simulink model "SolarTrackerSimulationModel"  (R2020a)
settings: Solver=FixedStepAuto  StartTime=0.0  StopTime=inf  RelTol=1e-3
libraries: sldrtlib x9, simulink x2
settings Model: SILPILModeSetting=veronly  EnablePacing=on  ExtModeTrigDuration=2  Creator=cstap  LastModifiedBy=dbhatia
settings OptimizationCC: EnhancedBackFolding=on  PassReuseOutputArgsAs=Individual arguments  ZeroExternalMemoryAtStartup=off  ZeroInternalMemoryAtStartup=off  MaxStackSize=64  OptimizeBlockOrder=speed  DifferentSizesBufferReuse=on  OptimizationCustomize=off  EfficientTunableParamExpr=on
settings DebuggingCC: ParameterTunabilityLossMsg=error
settings HardwareCC: ProdBitPerPointer=32  ProdBitPerSizeT=32  ProdBitPerPtrDiffT=32  ProdLargestAtomicInteger=Long  ProdLargestAtomicFloat=Double  ProdWordSize=32  ProdHWDeviceType=ARM Compatible->ARM Cortex
settings SFSimCC: MATLABDynamicMemAlloc=off
settings RTWCC: SystemTargetFile=ert.tlc  HardwareBoard=Arduino MKR1000  TLCOptions=-aInlineSetEventsForThisBaseRateFcn=TLC_FALSE -aSuppressMultiTaskScheduler=TLC_FALSE -aRateBasedStepFcn=1  TemplateMakefile=ert_default_tmf  Toolchain=Arduino ARM  BuildConfiguration=Faster Runs
settings CodeAppCC: ForceParamTrailComments=on  IgnoreCustomStorageClasses=off  OperatorAnnotations=on  SimulinkDataObjDesc=on  SFDataObjDesc=on  InsertBlockDesc=on
settings ERTTargetCC: SupportContinuousTime=on  SupportVariableSizeSignals=on  ExtModeStaticAllocSize=8192

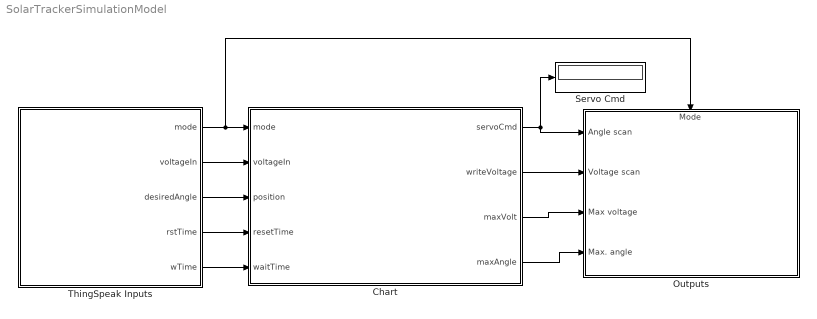
== system SolarTrackerSimulationModel ==
  Chart : Stateflow chart  TreatAsAtomicUnit=on
      settings: PortSchema="{\"entries\":[{\"content\":{\"sides\":[{\"content\":{\"connectorIds\":[\"In5\",\"In1\",\"In2\",\"In3\",\"In4\"]},\"type\":\"ConnectorPlacement.EquallySpacedRectSide\",\"uuid\":\"7460febf-f6e8-4dab-9ef6-8acf957c7b17\"},{\"content\":{\"connectorIds\":[\"Out1\",\"Out2\",\"Out3\",\"Out4\"],\"side\":\"RIGHT\"},\"type\":\"ConnectorPlacement.EquallySpacedRectSide\",\"uuid\":\"34f4fde0-3abd-4f83-b5ac-d115b7860e10\"},{\"content\":{\"connectorIds\":[],\"side\":\"TOP\"},\"type\":\"ConnectorPlacement.EquallySpacedRectSide\",\"uuid\":\"03c52414-b361-422d-a974-9760757eaedc\"}]},\"type\":\"ConnectorPlacement.EquallySpacedConnector\",\"uuid\":\"cf5b2fd0-3883-4494-a5b1-8c312db57bd7\"}],\"packageUris\":[\"http://schema.mathworks.com/mf0/Connector/19700101\"],\"version\":\"1.0\"}"
  Outputs : Subsystem
      settings: PortSchema="{\"entries\":[{\"content\":{\"sides\":[{\"content\":{\"connectorIds\":[\"In1\",\"In2\",\"In3\",\"In4\"]},\"type\":\"ConnectorPlacement.EquallySpacedRectSide\",\"uuid\":\"80b3db40-b16c-4fd7-bc95-d011d1dc8e0f\"},{\"content\":{\"connectorIds\":[],\"side\":\"RIGHT\"},\"type\":\"ConnectorPlacement.EquallySpacedRectSide\",\"uuid\":\"c08e910d-1728-45ea-85cd-9044765ba3b0\"},{\"content\":{\"connectorIds\":[\"In5\"],\"side\":\"TOP\"},\"type\":\"ConnectorPlacement.EquallySpacedRectSide\",\"uuid\":\"a6fb2687-566e-4921-9db4-7b726284379e\"}]},\"type\":\"ConnectorPlacement.EquallySpacedConnector\",\"uuid\":\"da0eea2f-bb34-402a-a1e4-ed3247ba3f26\"}],\"packageUris\":[\"http://schema.mathworks.com/mf0/Connector/19700101\"],\"version\":\"1.0\"}"
  Servo Cmd : Display
  ThingSpeak Inputs : Subsystem
  wires:
  ThingSpeak Inputs/1(mode) -> Outputs/5(Mode), Chart/5(mode)
  ThingSpeak Inputs/2(voltageIn) -> Chart/1(voltageIn)
  ThingSpeak Inputs/3(desiredAngle) -> Chart/2(position)
  ThingSpeak Inputs/4(rstTime) -> Chart/3(resetTime)
  ThingSpeak Inputs/5(wTime) -> Chart/4(waitTime)
  Chart/2(writeVoltage) -> Outputs/2(Voltage scan)
  Chart/3(maxVolt) -> Outputs/3(Max voltage)
  Chart/4(maxAngle) -> Outputs/4(Max. angle)
  Chart/1(servoCmd) -> Outputs/1(Angle scan), Servo Cmd/1

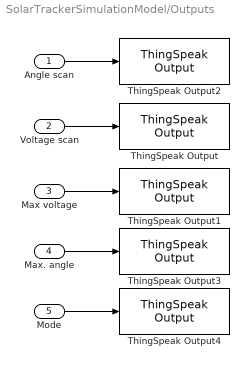
== system SolarTrackerSimulationModel/Outputs ==
  Angle scan : Inport
  Voltage scan : Inport  Port=2
  Max voltage : Inport  Port=3
  Max. angle : Inport  Port=4
  Mode : Inport  Port=5
  ThingSpeak Output : sldrtlib/Internet of Things/ThingSpeak Output  DrvAddress=1049171  DrvOptions=[1 10 77 88 84 86 78 50 89 78 70 66 88 88 75 72 71 55 97 112 105 46 116 104 105 110 103 115 112 101 97 107 46 99 111 109 0 0 0 0 0 0 0 0 0 0 0 0 0 0 0 0 0 0 0 0 0 0 0 0 0 0 0 0 0 0 0 0 0 0 0 0 0 0 0 0 0 0 0 0 0 0 0 0 0 0 0 0 0 0 0 0 0 0 0 0 0 0 0 0 0 0 0 0 0 0 0 0 0 0 0 0 0 0 0 0 0 0 0 0 0 0 0 0 0 0 0 0 0 0 0 0 0 0 0 0 0 0 0 0 0 0 0 0 0 0 0 0 0 0 0 0 0 0 0 0 0 0 0 0 0 0 0 0 0 0 0 0 0 0 0 0 0 0 0 0 0 0 0 0 0 0 0 0 0 0 0 0 0 0 0 0 0 0 0 0 0 0 0 0 0 0 0 0 0 0 0 0 0 0 0 0 0 0 0 0 0 0 0 0 0 0 0 0 0 0 0 0 0 0 0 0 0 0 0 0 0 0 0 0 0 0 0 0 0 0 0 0 0 0 0 0 0 0 0 0]  SampleTime=15  MaxMissedTicks=10  ShowMissedTicks=off  YieldWhenWaiting=off  ChannelFields=1  OptParam=0  InitialValue=[]  FinalValue=[]
      settings: SourceProductBaseCode=WT
  ThingSpeak Output1 : sldrtlib/Internet of Things/ThingSpeak Output  DrvAddress=1049171  DrvOptions=[1 10 77 88 84 86 78 50 89 78 70 66 88 88 75 72 71 55 97 112 105 46 116 104 105 110 103 115 112 101 97 107 46 99 111 109 0 0 0 0 0 0 0 0 0 0 0 0 0 0 0 0 0 0 0 0 0 0 0 0 0 0 0 0 0 0 0 0 0 0 0 0 0 0 0 0 0 0 0 0 0 0 0 0 0 0 0 0 0 0 0 0 0 0 0 0 0 0 0 0 0 0 0 0 0 0 0 0 0 0 0 0 0 0 0 0 0 0 0 0 0 0 0 0 0 0 0 0 0 0 0 0 0 0 0 0 0 0 0 0 0 0 0 0 0 0 0 0 0 0 0 0 0 0 0 0 0 0 0 0 0 0 0 0 0 0 0 0 0 0 0 0 0 0 0 0 0 0 0 0 0 0 0 0 0 0 0 0 0 0 0 0 0 0 0 0 0 0 0 0 0 0 0 0 0 0 0 0 0 0 0 0 0 0 0 0 0 0 0 0 0 0 0 0 0 0 0 0 0 0 0 0 0 0 0 0 0 0 0 0 0 0 0 0 0 0 0 0 0 0 0 0 0 0 0 0]  SampleTime=15  MaxMissedTicks=10  ShowMissedTicks=off  YieldWhenWaiting=off  ChannelFields=3  OptParam=0  InitialValue=[]  FinalValue=[]
      settings: SourceProductBaseCode=WT
  ThingSpeak Output2 : sldrtlib/Internet of Things/ThingSpeak Output  DrvAddress=1049171  DrvOptions=[1 10 77 88 84 86 78 50 89 78 70 66 88 88 75 72 71 55 97 112 105 46 116 104 105 110 103 115 112 101 97 107 46 99 111 109 0 0 0 0 0 0 0 0 0 0 0 0 0 0 0 0 0 0 0 0 0 0 0 0 0 0 0 0 0 0 0 0 0 0 0 0 0 0 0 0 0 0 0 0 0 0 0 0 0 0 0 0 0 0 0 0 0 0 0 0 0 0 0 0 0 0 0 0 0 0 0 0 0 0 0 0 0 0 0 0 0 0 0 0 0 0 0 0 0 0 0 0 0 0 0 0 0 0 0 0 0 0 0 0 0 0 0 0 0 0 0 0 0 0 0 0 0 0 0 0 0 0 0 0 0 0 0 0 0 0 0 0 0 0 0 0 0 0 0 0 0 0 0 0 0 0 0 0 0 0 0 0 0 0 0 0 0 0 0 0 0 0 0 0 0 0 0 0 0 0 0 0 0 0 0 0 0 0 0 0 0 0 0 0 0 0 0 0 0 0 0 0 0 0 0 0 0 0 0 0 0 0 0 0 0 0 0 0 0 0 0 0 0 0 0 0 0 0 0 0]  SampleTime=15  MaxMissedTicks=10  ShowMissedTicks=off  YieldWhenWaiting=off  ChannelFields=2  OptParam=0  InitialValue=[]  FinalValue=[]
      settings: SourceProductBaseCode=WT
  ThingSpeak Output3 : sldrtlib/Internet of Things/ThingSpeak Output  DrvAddress=1049171  DrvOptions=[1 10 77 88 84 86 78 50 89 78 70 66 88 88 75 72 71 55 97 112 105 46 116 104 105 110 103 115 112 101 97 107 46 99 111 109 0 0 0 0 0 0 0 0 0 0 0 0 0 0 0 0 0 0 0 0 0 0 0 0 0 0 0 0 0 0 0 0 0 0 0 0 0 0 0 0 0 0 0 0 0 0 0 0 0 0 0 0 0 0 0 0 0 0 0 0 0 0 0 0 0 0 0 0 0 0 0 0 0 0 0 0 0 0 0 0 0 0 0 0 0 0 0 0 0 0 0 0 0 0 0 0 0 0 0 0 0 0 0 0 0 0 0 0 0 0 0 0 0 0 0 0 0 0 0 0 0 0 0 0 0 0 0 0 0 0 0 0 0 0 0 0 0 0 0 0 0 0 0 0 0 0 0 0 0 0 0 0 0 0 0 0 0 0 0 0 0 0 0 0 0 0 0 0 0 0 0 0 0 0 0 0 0 0 0 0 0 0 0 0 0 0 0 0 0 0 0 0 0 0 0 0 0 0 0 0 0 0 0 0 0 0 0 0 0 0 0 0 0 0 0 0 0 0 0 0]  SampleTime=15  MaxMissedTicks=10  ShowMissedTicks=off  YieldWhenWaiting=off  ChannelFields=4  OptParam=0  InitialValue=[]  FinalValue=[]
      settings: SourceProductBaseCode=WT
  ThingSpeak Output4 : sldrtlib/Internet of Things/ThingSpeak Output  DrvAddress=1049171  DrvOptions=[1 10 77 88 84 86 78 50 89 78 70 66 88 88 75 72 71 55 97 112 105 46 116 104 105 110 103 115 112 101 97 107 46 99 111 109 0 0 0 0 0 0 0 0 0 0 0 0 0 0 0 0 0 0 0 0 0 0 0 0 0 0 0 0 0 0 0 0 0 0 0 0 0 0 0 0 0 0 0 0 0 0 0 0 0 0 0 0 0 0 0 0 0 0 0 0 0 0 0 0 0 0 0 0 0 0 0 0 0 0 0 0 0 0 0 0 0 0 0 0 0 0 0 0 0 0 0 0 0 0 0 0 0 0 0 0 0 0 0 0 0 0 0 0 0 0 0 0 0 0 0 0 0 0 0 0 0 0 0 0 0 0 0 0 0 0 0 0 0 0 0 0 0 0 0 0 0 0 0 0 0 0 0 0 0 0 0 0 0 0 0 0 0 0 0 0 0 0 0 0 0 0 0 0 0 0 0 0 0 0 0 0 0 0 0 0 0 0 0 0 0 0 0 0 0 0 0 0 0 0 0 0 0 0 0 0 0 0 0 0 0 0 0 0 0 0 0 0 0 0 0 0 0 0 0 0]  SampleTime=15  MaxMissedTicks=10  ShowMissedTicks=off  YieldWhenWaiting=off  ChannelFields=5  OptParam=0  InitialValue=[]  FinalValue=[]
      settings: SourceProductBaseCode=WT
  wires:
  Voltage scan/1 -> ThingSpeak Output/1
  Angle scan/1 -> ThingSpeak Output2/1
  Max voltage/1 -> ThingSpeak Output1/1
  Max. angle/1 -> ThingSpeak Output3/1
  Mode/1 -> ThingSpeak Output4/1

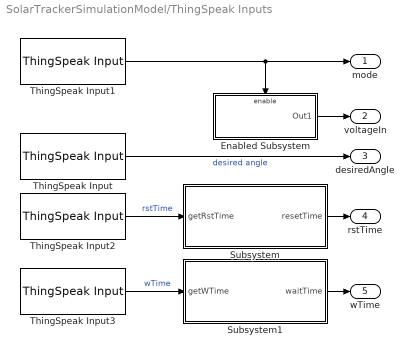
== system SolarTrackerSimulationModel/ThingSpeak Inputs ==
  Enabled Subsystem : Subsystem  TreatAsAtomicUnit=on
  Subsystem : Subsystem
  Subsystem1 : Subsystem
  ThingSpeak Input : sldrtlib/Internet of Things/ThingSpeak Input  DrvAddress=1049139  DrvOptions=[0 1 84 52 67 75 85 73 73 71 66 66 69 84 80 70 66 68 97 112 105 46 116 104 105 110 103 115 112 101 97 107 46 99 111 109 0 0 0 0 0 0 0 0 0 0 0 0 0 0 0 0 0 0 0 0 0 0 0 0 0 0 0 0 0 0 0 0 0 0 0 0 0 0 0 0 0 0 0 0 0 0 0 0 0 0 0 0 0 0 0 0 0 0 0 0 0 0 0 0 0 0 0 0 0 0 0 0 0 0 0 0 0 0 0 0 0 0 0 0 0 0 0 0 0 0 0 0 0 0 0 0 0 0 0 0 0 0 0 0 0 0 0 0 0 0 0 0 0 0 0 0 0 0 0 0 0 0 0 0 0 0 0 0 0 0 0 0 0 0 0 0 0 0 0 0 0 0 0 0 0 0 0 0 0 0 0 0 0 0 0 0 0 0 0 0 0 0 0 0 0 0 0 0 0 0 0 0 0 0 0 0 0 0 0 0 0 0 0 0 0 0 0 0 0 0 0 0 0 0 0 0 0 0 0 0 0 0 0 0 0 0 0 0 0 0 0 0 0 0 0 0 0 0 0 0]  SampleTime=0  MaxMissedTicks=10  ShowMissedTicks=off  YieldWhenWaiting=off  ChannelFields=2  OptParam=0  DataTypeStr=double
      settings: SourceProductBaseCode=WT
  ThingSpeak Input1 : sldrtlib/Internet of Things/ThingSpeak Input  DrvAddress=1049139  DrvOptions=[0 1 84 52 67 75 85 73 73 71 66 66 69 84 80 70 66 68 97 112 105 46 116 104 105 110 103 115 112 101 97 107 46 99 111 109 0 0 0 0 0 0 0 0 0 0 0 0 0 0 0 0 0 0 0 0 0 0 0 0 0 0 0 0 0 0 0 0 0 0 0 0 0 0 0 0 0 0 0 0 0 0 0 0 0 0 0 0 0 0 0 0 0 0 0 0 0 0 0 0 0 0 0 0 0 0 0 0 0 0 0 0 0 0 0 0 0 0 0 0 0 0 0 0 0 0 0 0 0 0 0 0 0 0 0 0 0 0 0 0 0 0 0 0 0 0 0 0 0 0 0 0 0 0 0 0 0 0 0 0 0 0 0 0 0 0 0 0 0 0 0 0 0 0 0 0 0 0 0 0 0 0 0 0 0 0 0 0 0 0 0 0 0 0 0 0 0 0 0 0 0 0 0 0 0 0 0 0 0 0 0 0 0 0 0 0 0 0 0 0 0 0 0 0 0 0 0 0 0 0 0 0 0 0 0 0 0 0 0 0 0 0 0 0 0 0 0 0 0 0 0 0 0 0 0 0]  SampleTime=0  MaxMissedTicks=10  ShowMissedTicks=off  YieldWhenWaiting=off  ChannelFields=1  OptParam=0  DataTypeStr=double
      settings: SourceProductBaseCode=WT
  ThingSpeak Input2 : sldrtlib/Internet of Things/ThingSpeak Input  DrvAddress=1049139  DrvOptions=[0 1 84 52 67 75 85 73 73 71 66 66 69 84 80 70 66 68 97 112 105 46 116 104 105 110 103 115 112 101 97 107 46 99 111 109 0 0 0 0 0 0 0 0 0 0 0 0 0 0 0 0 0 0 0 0 0 0 0 0 0 0 0 0 0 0 0 0 0 0 0 0 0 0 0 0 0 0 0 0 0 0 0 0 0 0 0 0 0 0 0 0 0 0 0 0 0 0 0 0 0 0 0 0 0 0 0 0 0 0 0 0 0 0 0 0 0 0 0 0 0 0 0 0 0 0 0 0 0 0 0 0 0 0 0 0 0 0 0 0 0 0 0 0 0 0 0 0 0 0 0 0 0 0 0 0 0 0 0 0 0 0 0 0 0 0 0 0 0 0 0 0 0 0 0 0 0 0 0 0 0 0 0 0 0 0 0 0 0 0 0 0 0 0 0 0 0 0 0 0 0 0 0 0 0 0 0 0 0 0 0 0 0 0 0 0 0 0 0 0 0 0 0 0 0 0 0 0 0 0 0 0 0 0 0 0 0 0 0 0 0 0 0 0 0 0 0 0 0 0 0 0 0 0 0 0]  SampleTime=0  MaxMissedTicks=10  ShowMissedTicks=off  YieldWhenWaiting=off  ChannelFields=3  OptParam=0  DataTypeStr=double
      settings: SourceProductBaseCode=WT
  ThingSpeak Input3 : sldrtlib/Internet of Things/ThingSpeak Input  DrvAddress=1049139  DrvOptions=[0 1 84 52 67 75 85 73 73 71 66 66 69 84 80 70 66 68 97 112 105 46 116 104 105 110 103 115 112 101 97 107 46 99 111 109 0 0 0 0 0 0 0 0 0 0 0 0 0 0 0 0 0 0 0 0 0 0 0 0 0 0 0 0 0 0 0 0 0 0 0 0 0 0 0 0 0 0 0 0 0 0 0 0 0 0 0 0 0 0 0 0 0 0 0 0 0 0 0 0 0 0 0 0 0 0 0 0 0 0 0 0 0 0 0 0 0 0 0 0 0 0 0 0 0 0 0 0 0 0 0 0 0 0 0 0 0 0 0 0 0 0 0 0 0 0 0 0 0 0 0 0 0 0 0 0 0 0 0 0 0 0 0 0 0 0 0 0 0 0 0 0 0 0 0 0 0 0 0 0 0 0 0 0 0 0 0 0 0 0 0 0 0 0 0 0 0 0 0 0 0 0 0 0 0 0 0 0 0 0 0 0 0 0 0 0 0 0 0 0 0 0 0 0 0 0 0 0 0 0 0 0 0 0 0 0 0 0 0 0 0 0 0 0 0 0 0 0 0 0 0 0 0 0 0 0]  SampleTime=0  MaxMissedTicks=10  ShowMissedTicks=off  YieldWhenWaiting=off  ChannelFields=4  OptParam=0  DataTypeStr=double
      settings: SourceProductBaseCode=WT
  mode : Outport
  voltageIn : Outport  Port=2
  desiredAngle : Outport  Port=3
  rstTime : Outport  Port=4
  wTime : Outport  Port=5
  wires:
  ThingSpeak Input3/1 -> Subsystem1/1(getWTime)  "wTime"
  ThingSpeak Input1/1 -> mode/1, Enabled Subsystem/Enable
  ThingSpeak Input2/1 -> Subsystem/1(getRstTime)  "rstTime"
  Enabled Subsystem/1(Out1) -> voltageIn/1
  ThingSpeak Input/1 -> desiredAngle/1  "desired angle"
  Subsystem/1(resetTime) -> rstTime/1
  Subsystem1/1(waitTime) -> wTime/1

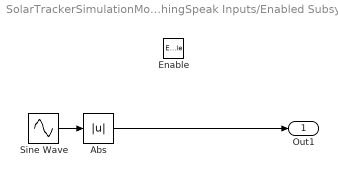
== system SolarTrackerSimulationModel/ThingSpeak Inputs/Enabled Subsystem ==
  Enable : EnablePort  StatesWhenEnabling=reset
  Abs : Abs
  Sine Wave : Sin  Amplitude=3.4  Frequency=0.01  SampleTime=0
  Out1 : Outport
  wires:
  Abs/1 -> Out1/1
  Sine Wave/1 -> Abs/1

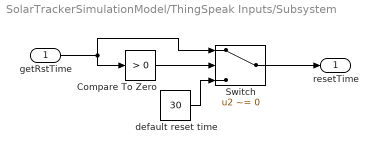
== system SolarTrackerSimulationModel/ThingSpeak Inputs/Subsystem ==
  getRstTime : Inport  OutDataTypeStr=double
  Compare To Zero : simulink/Logic and Bit Operations/Compare To Zero  relop=>  OutDataTypeStr=boolean
  Switch : Switch  Criteria=u2 ~= 0
  default reset time : Constant  Value=30  SampleTime=0
  resetTime : Outport  OutDataTypeStr=double
  wires:
  Compare To Zero/1 -> Switch/2
  default reset time/1 -> Switch/3
  getRstTime/1 -> Switch/1, Compare To Zero/1
  Switch/1 -> resetTime/1

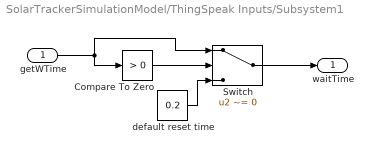
== system SolarTrackerSimulationModel/ThingSpeak Inputs/Subsystem1 ==
  getWTime : Inport  OutDataTypeStr=double
  Compare To Zero : simulink/Logic and Bit Operations/Compare To Zero  relop=>  OutDataTypeStr=boolean
  Switch : Switch  Criteria=u2 ~= 0
  default reset time : Constant  Value=0.2  SampleTime=0
  waitTime : Outport  OutDataTypeStr=double
  wires:
  Compare To Zero/1 -> Switch/2
  default reset time/1 -> Switch/3
  getWTime/1 -> Switch/1, Compare To Zero/1
  Switch/1 -> waitTime/1

== stateflow chart SolarTrackerSimulationModel/Chart ==
  settings: updateMethod=DISCRETE  sampleTime=0.1
  state GoToPosition
    servoCmd = position;
    writeVoltage=voltageIn;
  state ScanAndGoToMaxVoltage
    state ResetPosition
      servoCmd = 0;
      voltage = zeros(1,181);
    state ScanVoltages
      servoCmd = angleRange(i);
      voltage(i) = voltageIn;
      writeVoltage = voltage(i);
    state Increment
      entry: i = i + 1;
    state GoToMaxVoltage
      [maxVolt,maxVoltAngle] = max(voltage);
      servoCmd = angleRange(maxVoltAngle);
      maxAngle = servoCmd;
      writeVoltage=voltageIn;
    (default) -> ResetPosition : {angleRange = 0 :180;}
    GoToMaxVoltage -> ResetPosition : after(resetTime,sec)
    ResetPosition -> ScanVoltages : {i = 1;}
    ScanVoltages -> Increment [order 1] : [i < 181]
    Increment -> ScanVoltages : after(waitTime,sec)
    ScanVoltages -> GoToMaxVoltage [order 2] : [i==181]
  (default) -> GoToPosition
  GoToPosition -> ScanAndGoToMaxVoltage : [mode==1]
  ScanAndGoToMaxVoltage -> GoToPosition : [mode==0]
  data: voltageIn input; position input; servoCmd output; writeVoltage output; maxVolt output; maxAngle output; voltage local; i local; maxVoltAngle local; resetTime input; waitTime input; mode input; angleRange local
